simulink model "assignment_1_a"  (R2021a)
settings: Solver=VariableStepAuto  StartTime=0.0  StopTime=10  RelTol=1e-3
undefined symbols (not defined in the file): c1, c2, k1, k2, m1, m2
settings Model: Creator=vedan  LastModifiedBy=vedan

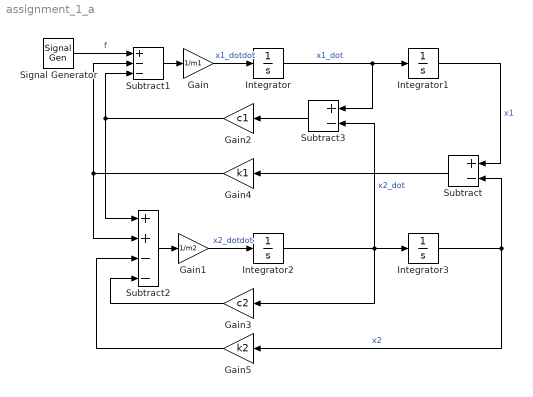
== system assignment_1_a ==
  Gain : Gain  Gain=1/m1
  Gain1 : Gain  Gain=1/m2
  Gain2 : Gain  Gain=c1
  Gain3 : Gain  Gain=c2
  Gain4 : Gain  Gain=k1
  Gain5 : Gain  Gain=k2
  Integrator{,1..3} (4 alike) : Integrator
  Signal Generator : SignalGenerator  Units=rad/sec
  Subtract : Sum  Inputs=+-
  Subtract1 : Sum  Inputs=+--
  Subtract2 : Sum  Inputs=++--
  Subtract3 : Sum  Inputs=+-
  wires:
  Gain/1 -> Integrator/1  "x1_dotdot"
  Integrator/1 -> Subtract3/1, Integrator1/1  "x1_dot"
  Integrator1/1 -> Subtract/1  "x1"
  Gain1/1 -> Integrator2/1  "x2_dotdot"
  Integrator2/1 -> Subtract3/2, Gain3/1, Integrator3/1  "x2_dot"
  Integrator3/1 -> Subtract/2, Gain5/1  "x2"
  Subtract/1 -> Gain4/1
  Subtract1/1 -> Gain/1
  Subtract2/1 -> Gain1/1
  Gain3/1 -> Subtract2/4
  Gain5/1 -> Subtract2/3
  Gain4/1 -> Subtract1/2, Subtract2/2
  Subtract3/1 -> Gain2/1
  Gain2/1 -> Subtract1/3, Subtract2/1
  Signal Generator/1 -> Subtract1/1  "f"
